simulink model "Simulation and Modelling 2st model"  (R2023a)
settings: Solver=VariableStepAuto  StartTime=0.0  StopTime=1000  RelTol=1e-3
undefined symbols (not defined in the file): m, n
settings Model: Creator=trian  LastModifiedBy=trian

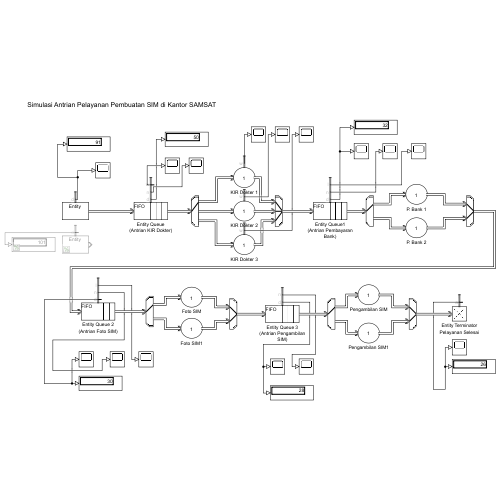
[thumbnail: Simulink's stored preview of the top-level diagram]
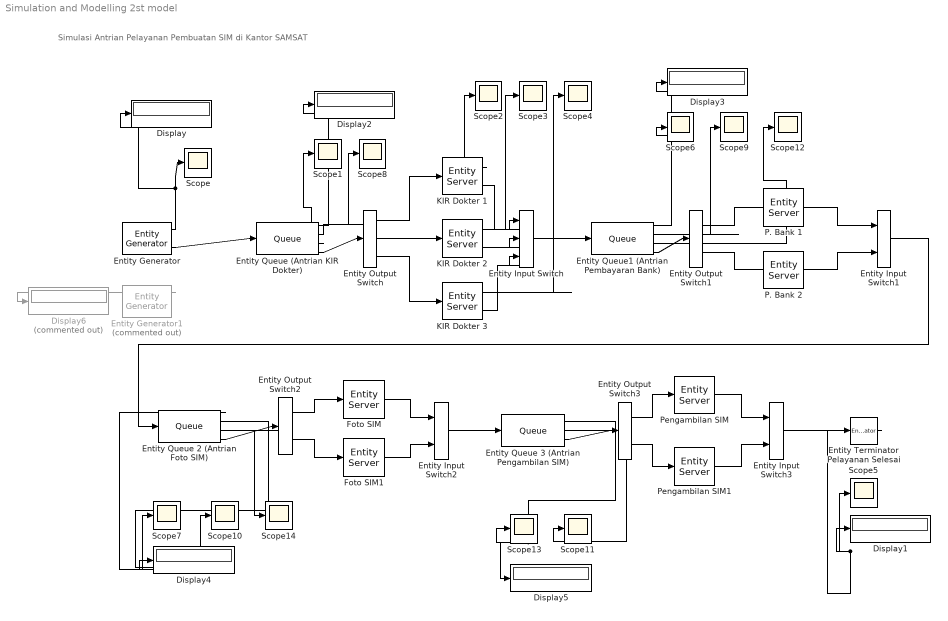
== system Simulation and Modelling 2st model ==
  note: Simulasi Antrian Pelayanan Pembuatan SIM di Kantor SAMSAT
  Display{,1..5} (6 alike) : Display
  Display6 : Display  Commented=on
  Entity Input Switch : EntityInputSwitch  InputPortMessageModes=m,m,m  OutputPortMessageModes=m  NumberInputPorts=3
      settings: InputPortMap=u1,u2,u3
  Entity Input Switch1 : EntityInputSwitch  InputPortMessageModes=m,m  OutputPortMessageModes=m
  Entity Input Switch2 : EntityInputSwitch  InputPortMessageModes=m,m  OutputPortMessageModes=m
  Entity Input Switch3 : EntityInputSwitch  InputPortMessageModes=m,m  OutputPortMessageModes=m
  Entity Output Switch : EntityOutputSwitch  InputPortMessageModes=m  OutputPortMessageModes=m,m,m  NumberOutputPorts=3  SwitchAttributeName=Attribute1
      settings: OutputPortMap=o0,o1,o2
  Entity Output Switch1 : EntityOutputSwitch  InputPortMessageModes=m  OutputPortMessageModes=m,m  SwitchAttributeName=Attribute1
  Entity Output Switch2 : EntityOutputSwitch  InputPortMessageModes=m  OutputPortMessageModes=m,m  SwitchAttributeName=Attribute1
  Entity Output Switch3 : EntityOutputSwitch  InputPortMessageModes=m  OutputPortMessageModes=m,m  SwitchAttributeName=Attribute1
  Entity Generator : EntityGenerator  OutputPortMessageModes=n,m  TimeSource=MATLAB action  IntergenerationTimeAction=|  NumberEntitiesDeparted=on  EntityType=Structured  EntityTypeName=Entity
      | mean = 10;
      | dt = -mean*log(1-rand());
      settings: OutputPortMap=o0,o3
  Entity Generator1 : EntityGenerator  Commented=on  OutputPortMessageModes=n,m  TimeSource=MATLAB action  IntergenerationTimeAction=dt = 10;  NumberEntitiesDeparted=on  EntityType=Structured  EntityTypeName=Entity
      settings: OutputPortMap=o0,o3
  Entity Queue (Antrian KIR Dokter) : Queue  InputPortMessageModes=m  OutputPortMessageModes=n,n,n,m  Capacity=inf  NumberEntitiesDeparted=on  NumberEntitiesInBlock=on  AverageWait=on
      settings: OutputPortMap=o0,o1,o2,o5
  Entity Queue 2 (Antrian Foto SIM) : Queue  InputPortMessageModes=m  OutputPortMessageModes=n,n,n,m  Capacity=inf  NumberEntitiesDeparted=on  NumberEntitiesInBlock=on  AverageQueueLength=on
      settings: OutputPortMap=o0,o1,o3,o5
  Entity Queue 3 (Antrian Pengambilan SIM) : Queue  InputPortMessageModes=m  OutputPortMessageModes=n,n,m  Capacity=inf  NumberEntitiesDeparted=on  NumberEntitiesInBlock=on
      settings: OutputPortMap=o0,o1,o5
  Entity Queue1 (Antrian Pembayaran Bank) : Queue  InputPortMessageModes=m  OutputPortMessageModes=n,n,n,m  Capacity=inf  NumberEntitiesDeparted=on  NumberEntitiesInBlock=on  AverageQueueLength=on
      settings: OutputPortMap=o0,o1,o3,o5
  Entity Terminator Pelayanan Selesai : EntityTerminator  InputPortMessageModes=m  NumberEntitiesArrived=on
      settings: OutputPortMap=o0
  Foto SIM : EntityServer  InputPortMessageModes=m  OutputPortMessageModes=m  Capacity=1  ServiceTimeValue=60.0
  Foto SIM1 : EntityServer  InputPortMessageModes=m  OutputPortMessageModes=m  Capacity=1  ServiceTimeValue=60.0
  KIR Dokter 1 : EntityServer  InputPortMessageModes=m  OutputPortMessageModes=n,m  Capacity=1  ServiceTimeValue=60.0  AverageWait=on
      settings: OutputPortMap=o4,o9
  KIR Dokter 2 : EntityServer  InputPortMessageModes=m  OutputPortMessageModes=n,m  Capacity=1  ServiceTimeValue=60  AverageWait=on
      settings: OutputPortMap=o4,o9
  KIR Dokter 3 : EntityServer  InputPortMessageModes=m  OutputPortMessageModes=n,m  Capacity=1  ServiceTimeValue=60  AverageWait=on
      settings: OutputPortMap=o4,o9
  P. Bank 1 : EntityServer  InputPortMessageModes=m  OutputPortMessageModes=m  Capacity=1  ServiceTimeValue=60.0
  P. Bank 2 : EntityServer  InputPortMessageModes=m  OutputPortMessageModes=m  Capacity=1  ServiceTimeValue=60.0
  Pengambilan SIM : EntityServer  InputPortMessageModes=m  OutputPortMessageModes=m  Capacity=1  ServiceTimeValue=60.0
  Pengambilan SIM1 : EntityServer  InputPortMessageModes=m  OutputPortMessageModes=m  Capacity=1  ServiceTimeValue=60.0
  Scope{,1..14} (15 alike) : Scope
  wires:
  Entity Queue (Antrian KIR Dokter)/4 -> Entity Output Switch/1
  Entity Output Switch/1 -> KIR Dokter 1/1
  Entity Output Switch/2 -> KIR Dokter 2/1
  Entity Output Switch/3 -> KIR Dokter 3/1
  KIR Dokter 1/2 -> Entity Input Switch/1
  KIR Dokter 2/2 -> Entity Input Switch/2
  KIR Dokter 3/2 -> Entity Input Switch/3
  Entity Input Switch/1 -> Entity Queue1 (Antrian Pembayaran Bank)/1
  Entity Queue1 (Antrian Pembayaran Bank)/4 -> Entity Output Switch1/1
  Entity Output Switch1/1 -> P. Bank 1/1
  Entity Output Switch1/2 -> P. Bank 2/1
  P. Bank 1/1 -> Entity Input Switch1/1
  P. Bank 2/1 -> Entity Input Switch1/2
  Entity Input Switch1/1 -> Entity Queue 2 (Antrian Foto SIM)/1
  Entity Queue (Antrian KIR Dokter)/3 -> Scope1/1
  Entity Terminator Pelayanan Selesai/1 -> Scope5/1, Display1/1
  Entity Queue1 (Antrian Pembayaran Bank)/1 -> Scope6/1, Display3/1
  KIR Dokter 1/1 -> Scope2/1
  KIR Dokter 2/1 -> Scope3/1
  KIR Dokter 3/1 -> Scope4/1
  Entity Queue (Antrian KIR Dokter)/2 -> Scope8/1
  Entity Queue1 (Antrian Pembayaran Bank)/2 -> Scope9/1
  Entity Queue 2 (Antrian Foto SIM)/2 -> Scope10/1
  Entity Queue 3 (Antrian Pengambilan SIM)/2 -> Scope11/1
  Entity Generator/1 -> Scope/1, Display/1
  Entity Queue (Antrian KIR Dokter)/1 -> Display2/1
  Entity Queue 2 (Antrian Foto SIM)/1 -> Scope7/1, Display4/1
  Entity Queue 3 (Antrian Pengambilan SIM)/1 -> Display5/1, Scope13/1
  Entity Queue 2 (Antrian Foto SIM)/4 -> Entity Output Switch2/1
  Entity Output Switch2/1 -> Foto SIM/1
  Entity Output Switch2/2 -> Foto SIM1/1
  Foto SIM/1 -> Entity Input Switch2/1
  Foto SIM1/1 -> Entity Input Switch2/2
  Entity Input Switch2/1 -> Entity Queue 3 (Antrian Pengambilan SIM)/1
  Entity Queue 3 (Antrian Pengambilan SIM)/3 -> Entity Output Switch3/1
  Entity Output Switch3/1 -> Pengambilan SIM/1
  Entity Output Switch3/2 -> Pengambilan SIM1/1
  Pengambilan SIM/1 -> Entity Input Switch3/1
  Pengambilan SIM1/1 -> Entity Input Switch3/2
  Entity Input Switch3/1 -> Entity Terminator Pelayanan Selesai/1
  Entity Generator1/1 -> Display6/1
  Entity Generator/2 -> Entity Queue (Antrian KIR Dokter)/1
  Entity Queue1 (Antrian Pembayaran Bank)/3 -> Scope12/1
  Entity Queue 2 (Antrian Foto SIM)/3 -> Scope14/1
